simulink library "atmoAttDisturbanceISS_sl"  (R2024b)
settings: Solver=VariableStepAuto  StartTime=0.0  StopTime=10.0  RelTol=1e-3
settings Model: Creator=gilbu
settings RTWCC: GPUComputeCapability=3.5

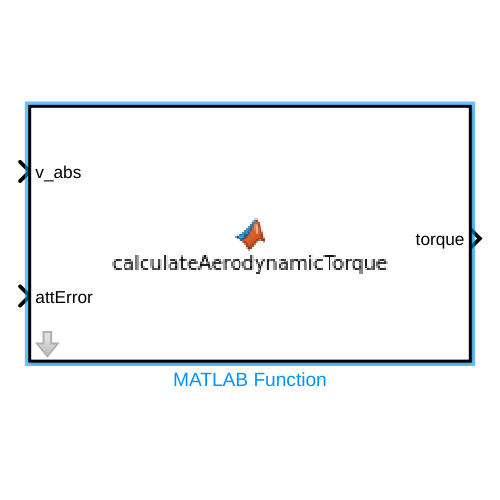
[thumbnail: Simulink's stored preview of the top-level diagram]
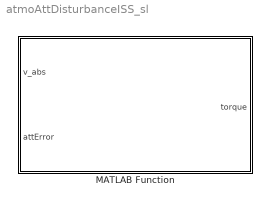
== system atmoAttDisturbanceISS_sl ==
  MATLAB Function : MATLAB Function  TreatAsAtomicUnit=on

== matlab function atmoAttDisturbanceISS_sl/MATLAB Function ==
  data: v_abs input; torque output; attError input
function torque = calculateAerodynamicTorque(v_abs, attError)
    % This function calculates the aerodynamic torque on the ISS
    % due to atmospheric drag, taking into account a pitching error.
    %
    % v_abs: The absolute velocity vector of the ISS in the ECI frame.
    % pitchingError: The pitching error in radians.
    % Author: Evan Sayer
    
    %----------------------------------------------------------------------
    % Air density at 400 km altitude in kg/m^3
    rho = 3e-12;
    
    % Pitching Error
    pitchingError = attError(2);
    
    % ISS dimensions in feet converted to meters
    length = 239 * 0.3048; % 239 ft to meters
    width = 356 * 0.3048; % 356 ft to meters
    height = 170 * 0.3048; % 170 ft to meters
    
    % Calculate cross-sectional area and effective area
    A = length * width*2/3; % Cross-sectional area in m^2
    A_p = A * cos(pitchingError); % Adjust area based on pitching error
    
    % Normal vector to the ISS surface accounting for pitching error
    normal_vector = [cos(pitchingError); 0; -sin(pitchingError)];
    
    % Calculate the magnitude of the absolute velocity
    v_abs_mag = norm(v_abs);
    
    % Project the absolute velocity onto the normal vector to get the component of velocity
    % that is perpendicular to the surface
    v_perpendicular = (dot(v_abs, normal_vector) / v_abs_mag) * v_abs;
    
    % Calculate the force due to aerodynamic drag in the direction opposite to the airflow
    f_aero = -rho * A_p * v_abs_mag * v_perpendicular;
    
    % The position vector from the center of pressure to the center of mass
    % r_cm is oriented along the drag axis and rotates with the pitching error
    r_cm = [(height / 2) * sin(pitchingError); 0; (height / 2) * cos(pitchingError)];
    
    % Calculate the torque using the cross product of r_cm and f_aero
    torque = cross(r_cm, f_aero);
end
